simulink model "CalclateFlyingSystem"  (R2016b)
settings: Solver=FixedStepAuto  StartTime=0.0  StopTime=10.0  RelTol=1e-3
settings Model: Creator=NEATdemo  LastModifiedBy=NEATdemo

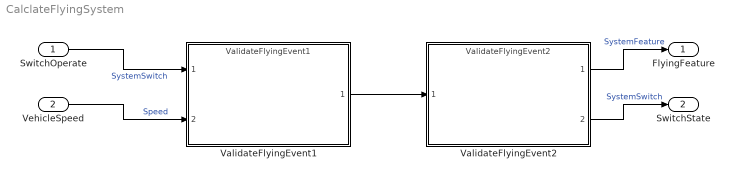
== system CalclateFlyingSystem ==
  SwitchOperate : Inport
      settings: AttributesFormatString=SystemSwitch
  VehicleSpeed : Inport  Port=2
      settings: AttributesFormatString=Speed
  ValidateFlyingEvent1 : ModelReference  ModelNameDialog=ValidateFlyingEvent1  SimulationMode=Normal  ModelReferenceVersion=1.6
  ValidateFlyingEvent2 : ModelReference  ModelNameDialog=ValidateFlyingEvent2  SimulationMode=Normal  ModelReferenceVersion=1.4
  FlyingFeature : Outport
      settings: AttributesFormatString=SystemFeature
  SwitchState : Outport  Port=2
      settings: AttributesFormatString=SystemSwitch
  wires:
  ValidateFlyingEvent1/1 -> ValidateFlyingEvent2/1
  SwitchOperate/1 -> ValidateFlyingEvent1/1  "SystemSwitch"
  VehicleSpeed/1 -> ValidateFlyingEvent1/2  "Speed"
  ValidateFlyingEvent2/2 -> SwitchState/1  "SystemSwitch"
  ValidateFlyingEvent2/1 -> FlyingFeature/1  "SystemFeature"
